simulink model "UD_model"  (R2021a)
settings: Solver=VariableStepAuto  StartTime=0.0  StopTime=2.5  MaxStep=1/60  RelTol=1e-3
PreLoadFcn:
  | load('parameters.mat');
values from neighbouring files (symbols this model uses):
  coulomb_omega = 0.001    [parameters.mat]
  Fc = 6.06272950939    [parameters.mat]
  gamma = 1.33283393094    [parameters.mat]
  Ku = 28.1361584072    [parameters.mat]
  omega0 = 11.3398469573    [parameters.mat]
libraries: vrlib x2
settings Model: EnablePacing=on  Creator=Patrick  LastModifiedBy=s143190
settings SolverCC: AlgebraicLoopSolver=TrustRegion
settings DataIOCC: ReturnWorkspaceOutputs=off
settings DebuggingCC: SFMachineParentedDataDiag=warning  ArithmeticOperatorsInVariantConditions=warning
settings SFSimCC: CustomCodeUndefinedFunction=UseInterfaceOnly

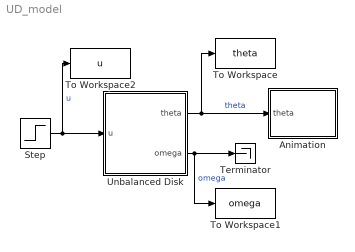
== system UD_model ==
  Animation : Subsystem
  Step : Step  Time=0  After=3  SampleTime=0.025
  Terminator : Terminator
  To Workspace : ToWorkspace  VariableName=theta  SaveFormat=Timeseries  SampleTime=-1
  To Workspace1 : ToWorkspace  VariableName=omega  SaveFormat=Timeseries  SampleTime=-1
  To Workspace2 : ToWorkspace  VariableName=u  SaveFormat=Timeseries  SampleTime=-1
  Unbalanced Disk : Subsystem  mask{theta_0=0, omega_0=0}
      mask prompts: theta_0 "Initial condition theta"; omega_0 "Initial condition omega"
      mask DialogControl Param Prompt: Parameters
      mask Display: image('UnbalancedDisk.jpg');
  wires:
  Step/1 -> To Workspace2/1, Unbalanced Disk/1(u)  "u"
  Unbalanced Disk/1(theta) -> To Workspace/1, Animation/1(theta)  "theta"
  Unbalanced Disk/2(omega) -> To Workspace1/1, Terminator/1  "omega"

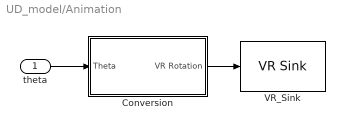
== system UD_model/Animation ==
  theta : Inport
  Conversion : Subsystem
  VR_Sink : vrlib/VR Sink  InstantiateOnLoad=on  SampleTime=-1  ViewEnable=on  RemoteChange=off  RemoteView=off  FieldsWritten=UD_Disc.rotation.4.1.1.double  WorldFileName=VR Model/UD_VR_World.wrl  AutoView=on  VideoDimensions=[]  AllowVariableSize=off
  wires:
  theta/1 -> Conversion/1(Theta)
  Conversion/1(VR Rotation) -> VR_Sink/1

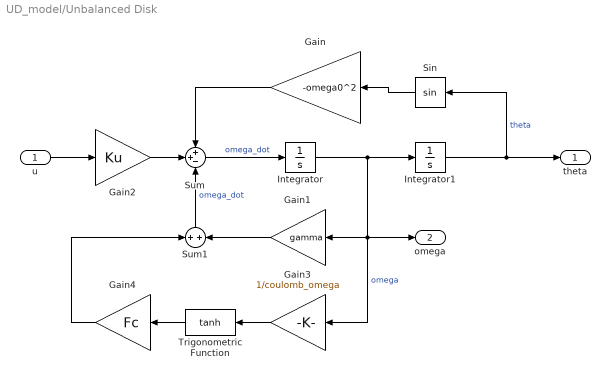
== system UD_model/Unbalanced Disk ==
  u : Inport
  Gain : Gain  Gain=-omega0^2
  Gain1 : Gain  Gain=gamma
  Gain2 : Gain  Gain=Ku
  Gain3 : Gain  Gain=1/coulomb_omega
  Gain4 : Gain  Gain=Fc
  Integrator : Integrator  InitialCondition=omega_0
  Integrator1 : Integrator  InitialCondition=theta_0
  Sin : Trigonometry
  Sum : Sum  Inputs=++-
  Sum1 : Sum
  Trigonometric Function : Trigonometry  Operator=tanh
  theta : Outport  VectorParamsAs1DForOutWhenUnconnected=off
  omega : Outport  Port=2  VectorParamsAs1DForOutWhenUnconnected=off
  wires:
  u/1 -> Gain2/1
  Sum/1 -> Integrator/1  "omega_dot"
  Sin/1 -> Gain/1
  Integrator/1 -> Gain3/1, omega/1, Gain1/1, Integrator1/1  "omega"
  Gain1/1 -> Sum1/2
  Gain2/1 -> Sum/2
  Integrator1/1 -> theta/1, Sin/1  "theta"
  Gain/1 -> Sum/1
  Gain3/1 -> Trigonometric Function/1
  Trigonometric Function/1 -> Gain4/1
  Gain4/1 -> Sum1/1
  Sum1/1 -> Sum/3  "omega_dot"

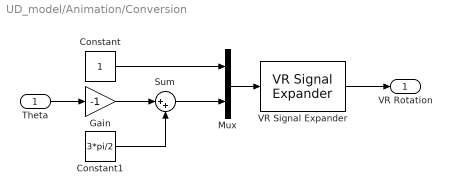
== system UD_model/Animation/Conversion ==
  Theta : Inport
  Constant : Constant
  Constant1 : Constant  Value=3*pi/2
  Gain : Gain  Gain=-1
  Mux : Mux  Inputs=2
  Sum : Sum  Inputs=|++
  VR Signal Expander : vrlib/VR Signal Expander  outwidth=4  outidx=[1 4]
  VR Rotation : Outport  VectorParamsAs1DForOutWhenUnconnected=off
  wires:
  Mux/1 -> VR Signal Expander/1
  Sum/1 -> Mux/2
  Gain/1 -> Sum/1
  Theta/1 -> Gain/1
  Constant1/1 -> Sum/2
  VR Signal Expander/1 -> VR Rotation/1
  Constant/1 -> Mux/1
